simulink model "sampleModel1923"  (R2023a)
settings: Solver=VariableStepAuto  StartTime=0.0  StopTime=10.0  RelTol=1e-3
libraries: hdlsllib x3, simulink x2
settings Model: Creator=user1  LastModifiedBy=user1

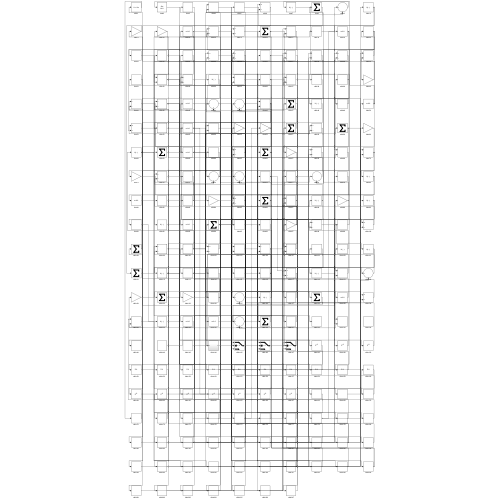
[thumbnail: Simulink's stored preview of the top-level diagram]
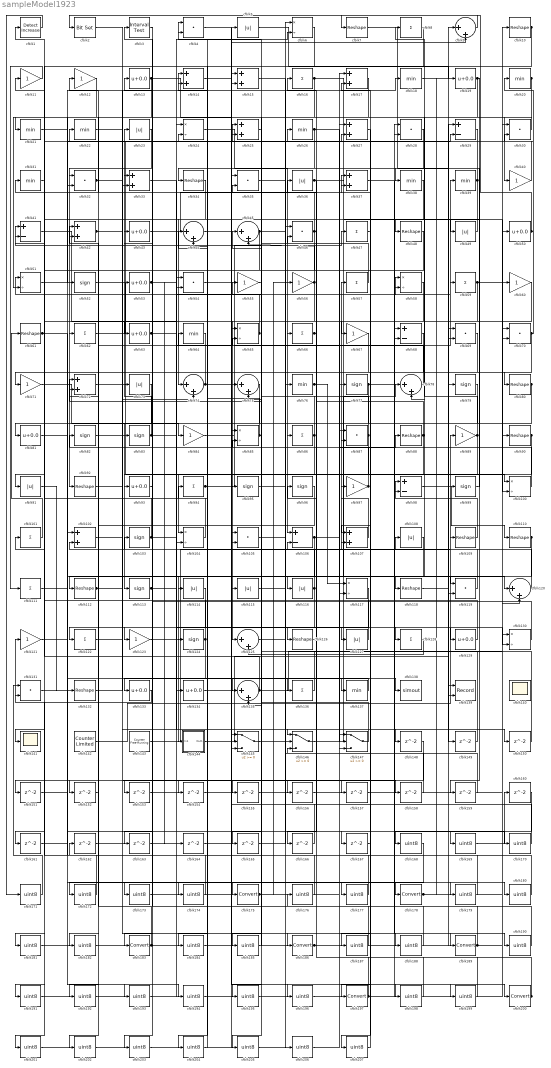
== system sampleModel1923 ==
  cfblk1 : simulink/Logic and Bit Operations/Detect Increase  vinit=0.0  OutDataTypeStr=boolean
      settings: LibrarySourceBlock=|
      | hdlsllib/Logic and Bit
      | Operations/Detect
      | Increase
  cfblk{7,10,34,48,61,80,88,90,92,109..110,112,118,126,132} (15 alike) : Reshape
  cfblk{6,24,51,58,65,85,100,104,117,130} (10 alike) : Product  Inputs=*/  RndMeth=Zero  SaturateOnIntegerOverflow=on
  cfblk{8,16,47,57,59,62,66,86,94,101,111,122,128,136} (14 alike) : Sum  Inputs=+
  cfblk{14..15,17,25,27,33,37,42,72,102,107} (11 alike) : Sum
  cfblk{52,77,79,82..83,95..96,99,103,113,124} (11 alike) : Signum
  cfblk{4,28,30,32,35,46,54,69..70,87,105,119,131} (13 alike) : DotProduct  OutDataTypeStr=Inherit: Inherit via internal rule
  cfblk{29,41,68,98,106} (5 alike) : Sum  Inputs=+-
  cfblk{5,23,36,49,73,91,108,114..116,127} (11 alike) : Abs  SaturateOnIntegerOverflow=off
  cfblk{11..12,40,55..56,60,67,71,84,89,97,121,123} (13 alike) : Gain
  cfblk{9,44..45,74..75,78,120,125,135} (9 alike) : Sum  Inputs=|++
  cfblk{13,19,43,50,53,63,81,93,129,133..134} (11 alike) : Bias  Bias=0.0  SaturateOnIntegerOverflow=off
  cfblk{18,20..22,26,31,38..39,64,76,137} (11 alike) : MinMax
  cfblk138 : ToWorkspace  VariableName=simout  SaveFormat=Timeseries  SampleTime=-1
  cfblk139 : Record  FileSettingsInternal="{\"entries\":[{\"content\":{\"excelSettings\":{\"content\":{},\"type\":\"Streamout.ExcelSettings\"}},\"type\":\"Streamout.FileSettingStorage\",\"uuid\":\"\"}],\"packageUris\":[\"http:\\/\\/schema.mathworks.com\\/mf0\\/streamout_blocks\\/R2020a\"],\"version\":\"1.0\"}"  Layout=[1 1]  SignalsInternal="{\"entries\":[{\"content\":{\"signals\":[{\"content\":{\"blockPath\":[],\"dimensions\":[1],\"domain\":\"\",\"lineColor\":\"#a2142f\",\"plots\":[1],\"port\":1,\"signalID\":5150,\"signalName\":\"XY Graph:1\"},\"type\":\"RecordBlkView.Signal\",\"uuid\":\"\"},{\"content\":{\"blockPath\":[],\"dimensions\":[1],\"domain\":\"\",\"lineColor\":\"#139fff\",\"plots\":[1],\"port\":2,\"signalID\":5153,\"signalName\":\"XY Graph:2\"},\"type\":\"RecordBlkView.Signal\",\"uuid\":\"\"}]},\"type\":\"RecordBlkView.InputSignals\",\"uuid\":\"\"}],\"packageUris\":[\"http:\\/\\/schema.mathworks.com\\/mf0\\/streamout_blocks\\/R2020a\"],\"version\":\"1.0\"}"  VisualizationBindings="{\"xyplotplugin\":{\"info\":[{\"series\":[{\"bindingParametersList\":[{\"parameter\":\"X-Axis\",\"signalID\":5150,\"signalName\":\"XY Graph:1\"},{\"parameter\":\"Y-Axis\",\"signalID\":5153,\"signalName\":\"XY Graph:2\"}],\"seriesID\":52586}],\"subplotID\":1}]}}"  CompatibilityTag=XY  st=-1
  cfblk140 : Scope
      settings: Floating=on
  cfblk141 : Scope
  cfblk142 : hdlsllib/Sources/Counter Limited  uplimit=7  tsamp=-1
  cfblk143 : hdlsllib/Sources/Counter Free-Running  NumBits=16  tsamp=-1
  cfblk144 : Subsystem
      settings: LibrarySourceBlock=|
      | hdlsllib/Ports &
      | Subsystems/Subsystem
  cfblk145 : Switch  SaturateOnIntegerOverflow=off  InputSameDT=off
  cfblk146 : Switch  SaturateOnIntegerOverflow=off  InputSameDT=off
  cfblk147 : Switch  SaturateOnIntegerOverflow=off  InputSameDT=off
  cfblk{148..167} (20 alike) : Delay  SampleTime=1
  cfblk{168..174,176..177,179..182,184..185,187..188,190..196,198..199,201..207} (33 alike) : DataTypeConversion  OutDataTypeStr=uint8  SaturateOnIntegerOverflow=off  RndMeth=Floor
  cfblk{175,178,183,186,189,197,200} (7 alike) : DataTypeConversion  SaturateOnIntegerOverflow=off  RndMeth=Floor
  cfblk2 : simulink/Logic and Bit Operations/Bit Set  iBit=0
      settings: LibrarySourceBlock=|
      | hdlsllib/Logic and Bit
      | Operations/Bit Set
  cfblk3 : hdlsllib/Logic and Bit Operations/Interval Test  IntervalClosedRight=on  uplimit=0.5  IntervalClosedLeft=on  lowlimit=-0.5  OutDataTypeStr=boolean
  wires:
  cfblk124/1 -> cfblk53/1, cfblk163/1
  cfblk65/1 -> cfblk51/1, cfblk13/1
  cfblk53/1 -> cfblk129/1, cfblk164/1
  cfblk137/1 -> cfblk133/1
  cfblk94/1 -> cfblk39/1, cfblk196/1
  cfblk142/1 -> cfblk89/1
  cfblk146/1 -> cfblk78/1
  cfblk99/1 -> cfblk38/1
  cfblk24/1 -> cfblk106/1
  cfblk62/1 -> cfblk26/1
  cfblk123/1 -> cfblk109/1
  cfblk110/1 -> cfblk125/1, cfblk187/1
  cfblk16/1 -> cfblk119/1, cfblk182/1
  cfblk43/1 -> cfblk37/1
  cfblk69/1 -> cfblk78/2
  cfblk109/1 -> cfblk98/1
  cfblk83/1 -> cfblk23/1, cfblk58/2
  cfblk125/1 -> cfblk76/1
  cfblk90/1 -> cfblk104/1, cfblk136/1
  cfblk87/1 -> cfblk113/1, cfblk41/1
  cfblk12/1 -> cfblk51/2
  cfblk76/1 -> cfblk126/1, cfblk117/1
  cfblk7/1 -> cfblk69/1
  cfblk86/1 -> cfblk31/1, cfblk185/1
  cfblk56/1 -> cfblk115/1, cfblk45/2
  cfblk66/1 -> cfblk16/1, cfblk86/1
  cfblk91/1 -> cfblk132/1
  cfblk84/1 -> cfblk47/1
  cfblk108/1 -> cfblk112/1
  cfblk49/1 -> cfblk48/1
  cfblk98/1 -> cfblk110/1
  cfblk29/1 -> cfblk24/2
  cfblk50/1 -> cfblk7/1, cfblk20/1
  cfblk129/1 -> cfblk55/1
  cfblk133/1 -> cfblk121/1
  cfblk143/1 -> cfblk108/1
  cfblk130/1 -> cfblk43/1
  cfblk127/1 -> cfblk11/1
  cfblk23/1 -> cfblk92/1
  cfblk4/1 -> cfblk127/1
  cfblk58/1 -> cfblk141/1
  cfblk11/1 -> cfblk111/1
  cfblk71/1 -> cfblk84/1
  cfblk97/1 -> cfblk82/1, cfblk14/2
  cfblk20/1 -> cfblk40/1, cfblk32/1, cfblk159/1
  cfblk48/1 -> cfblk81/1
  cfblk128/1 -> cfblk125/2
  cfblk89/1 -> cfblk8/1, cfblk184/1
  cfblk9/1 -> cfblk2/1
  cfblk38/1 -> cfblk85/1
  cfblk106/1 -> cfblk144/1(In1), cfblk88/1
  cfblk144/1(Out1) -> cfblk99/1
  cfblk61/1 -> cfblk137/1, cfblk193/1
  cfblk80/1 -> cfblk114/1, cfblk107/1
  cfblk52/1 -> cfblk100/1
  cfblk46/1 -> cfblk62/1, cfblk104/2, cfblk66/1, cfblk12/1
  cfblk85/1 -> cfblk4/1, cfblk135/1
  cfblk112/1 -> cfblk116/1, cfblk188/1
  cfblk72/1 -> cfblk98/2
  cfblk35/1 -> cfblk178/1
  cfblk2/1 -> cfblk73/1
  cfblk44/1 -> cfblk186/1
  cfblk70/1 -> cfblk80/1, cfblk30/2, cfblk147/2
  cfblk25/1 -> cfblk65/1
  cfblk39/1 -> cfblk74/1, cfblk1/1
  cfblk147/1 -> cfblk4/2
  cfblk45/1 -> cfblk167/1, cfblk204/1
  cfblk73/1 -> cfblk93/1
  cfblk15/1 -> cfblk200/1
  cfblk54/1 -> cfblk189/1
  cfblk36/1 -> cfblk100/2, cfblk166/1
  cfblk51/1 -> cfblk134/1
  cfblk77/1 -> cfblk28/1, cfblk95/1
  cfblk119/1 -> cfblk72/1
  cfblk120/1 -> cfblk57/1
  cfblk101/1 -> cfblk61/1
  cfblk111/1 -> cfblk120/1
  cfblk30/1 -> cfblk21/1
  cfblk13/1 -> cfblk145/1, cfblk32/2
  cfblk96/1 -> cfblk122/1
  cfblk126/1 -> cfblk96/1
  cfblk47/1 -> cfblk67/1
  cfblk57/1 -> cfblk33/1
  cfblk116/1 -> cfblk94/1, cfblk123/1
  cfblk42/1 -> cfblk156/1, cfblk157/1
  cfblk59/1 -> cfblk90/1, cfblk117/2
  cfblk81/1 -> cfblk29/2
  cfblk102/1 -> cfblk175/1
  cfblk107/1 -> cfblk97/1
  cfblk132/1 -> cfblk74/2
  cfblk5/1 -> cfblk139/1
  cfblk27/1 -> cfblk197/1
  cfblk10/1 -> cfblk34/1, cfblk139/2
  cfblk135/1 -> cfblk10/1, cfblk101/1, cfblk25/2
  cfblk113/1 -> cfblk130/2, cfblk58/1
  cfblk40/1 -> cfblk22/1
  cfblk82/1 -> cfblk83/1
  cfblk32/1 -> cfblk146/1, cfblk169/1
  cfblk41/1 -> cfblk63/1
  cfblk103/1 -> cfblk6/2, cfblk119/2, cfblk41/2
  cfblk63/1 -> cfblk59/1, cfblk65/2
  cfblk92/1 -> cfblk18/1
  cfblk74/1 -> cfblk71/1, cfblk9/2
  cfblk8/1 -> cfblk33/2
  cfblk134/1 -> cfblk138/1
  cfblk19/1 -> cfblk118/1, cfblk49/1
  cfblk78/1 -> cfblk42/1
  cfblk100/1 -> cfblk25/1
  cfblk75/1 -> cfblk183/1
  cfblk104/1 -> cfblk42/2
  cfblk136/1 -> cfblk72/2
  cfblk26/1 -> cfblk128/1, cfblk146/2
  cfblk22/1 -> cfblk145/2
  cfblk6/1 -> cfblk91/1
  cfblk88/1 -> cfblk124/1, cfblk36/1
  cfblk21/1 -> cfblk52/1
  cfblk18/1 -> cfblk9/1
  cfblk121/1 -> cfblk14/1
  cfblk115/1 -> cfblk148/1
  cfblk118/1 -> cfblk149/1
  cfblk149/1 -> cfblk37/2
  cfblk33/1 -> cfblk150/1
  cfblk150/1 -> cfblk85/2
  cfblk34/1 -> cfblk151/1
  cfblk114/1 -> cfblk152/1
  cfblk93/1 -> cfblk153/1
  cfblk153/1 -> cfblk29/1
  cfblk122/1 -> cfblk154/1
  cfblk154/1 -> cfblk130/1
  cfblk117/1 -> cfblk155/1
  cfblk156/1 -> cfblk106/2
  cfblk157/1 -> cfblk107/2
  cfblk145/1 -> cfblk158/1
  cfblk158/1 -> cfblk46/1
  cfblk159/1 -> cfblk87/2
  cfblk31/1 -> cfblk161/1
  cfblk162/1 -> cfblk105/2
  cfblk163/1 -> cfblk24/1
  cfblk55/1 -> cfblk165/1
  cfblk165/1 -> cfblk6/1
  cfblk166/1 -> cfblk45/1
  cfblk160/1 -> cfblk168/1
  cfblk169/1 -> cfblk160/1
  cfblk131/1 -> cfblk170/1
  cfblk170/1 -> cfblk105/1
  cfblk1/1 -> cfblk171/1
  cfblk171/1 -> cfblk131/1
  cfblk168/1 -> cfblk172/1
  cfblk172/1 -> cfblk131/2
  cfblk3/1 -> cfblk173/1
  cfblk173/1 -> cfblk5/1
  cfblk28/1 -> cfblk174/1
  cfblk174/1 -> cfblk3/1
  cfblk175/1 -> cfblk147/3, cfblk56/1
  cfblk176/1 -> cfblk102/1
  cfblk151/1 -> cfblk177/1
  cfblk177/1 -> cfblk102/2
  cfblk178/1 -> cfblk30/1, cfblk19/1
  cfblk164/1 -> cfblk179/1
  cfblk179/1 -> cfblk35/1
  cfblk95/1 -> cfblk180/1
  cfblk180/1 -> cfblk35/2
  cfblk79/1 -> cfblk181/1
  cfblk181/1 -> cfblk69/2
  cfblk182/1 -> cfblk79/1
  cfblk183/1 -> cfblk162/1, cfblk120/2, cfblk145/3
  cfblk184/1 -> cfblk75/1
  cfblk185/1 -> cfblk75/2
  cfblk186/1 -> cfblk28/2, cfblk50/1
  cfblk187/1 -> cfblk44/1
  cfblk188/1 -> cfblk44/2
  cfblk189/1 -> cfblk135/2, cfblk103/1
  cfblk37/1 -> cfblk190/1
  cfblk190/1 -> cfblk54/1
  cfblk148/1 -> cfblk191/1
  cfblk191/1 -> cfblk54/2
  cfblk68/1 -> cfblk192/1
  cfblk192/1 -> cfblk70/1
  cfblk193/1 -> cfblk68/1
  cfblk161/1 -> cfblk194/1
  cfblk194/1 -> cfblk68/2
  cfblk60/1 -> cfblk195/1
  cfblk195/1 -> cfblk70/2
  cfblk196/1 -> cfblk60/1
  cfblk197/1 -> cfblk46/2, cfblk147/1
  cfblk14/1 -> cfblk198/1
  cfblk198/1 -> cfblk27/1
  cfblk155/1 -> cfblk199/1
  cfblk199/1 -> cfblk27/2
  cfblk200/1 -> cfblk176/1, cfblk146/3
  cfblk67/1 -> cfblk201/1
  cfblk201/1 -> cfblk15/1
  cfblk152/1 -> cfblk202/1
  cfblk202/1 -> cfblk15/2
  cfblk64/1 -> cfblk203/1
  cfblk203/1 -> cfblk77/1
  cfblk204/1 -> cfblk64/1
  cfblk17/1 -> cfblk205/1
  cfblk205/1 -> cfblk87/1
  cfblk105/1 -> cfblk206/1
  cfblk206/1 -> cfblk17/1
  cfblk167/1 -> cfblk207/1
  cfblk207/1 -> cfblk17/2

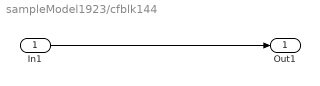
== system sampleModel1923/cfblk144 ==
  In1 : Inport
  Out1 : Outport
  wires:
  In1/1 -> Out1/1
